simulink model "altitude_from_pitch_loop"  (Simulink 7.4)
settings: Solver=ode45  StartTime=0.0  StopTime=100  RelTol=1e-3
values from neighbouring files (symbols this model uses):
  a_theta1 = den(2)    [computeGains.m]    (also in compute_tf_model.m = -rho*Va_trim^2 * cbar^2 * S_wing /(4*P.Jy) * P.C_M_q)
  a_theta2 = num(3)    [computeGains.m]    (also in compute_tf_model.m = -rho*Va_trim^2*cbar*S_wing/2/P.Jy*C_M_alpha)
  a_theta3 = rho*Va_trim^2*cbar*S_wing/2/P.Jy*C_M_delta_e    [compute_tf_model.m]
  delta_e_max = P.delta_e_max    [computeGains.m]
  P = varargin{5}    [my_mav_dynamics.m]
settings Model: Creator=beard  LastModifiedBy=beard

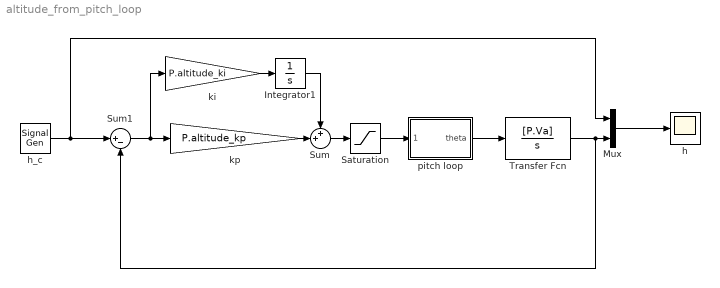
== system altitude_from_pitch_loop ==
  Integrator1 : Integrator
  Mux : Mux  Inputs=2
  Saturation : Saturate  UpperLimit=30*pi/180/P.K_theta_DC  LowerLimit=-30*pi/180/P.K_theta_DC  OutDataType=fixdt(1, 16)  OutScaling=2^0
  Sum : Sum  Inputs=++|  OutDataType=fixdt(1, 16)  OutScaling=2^0
  Sum1 : Sum  Inputs=|+-  OutDataType=fixdt(1, 16)  OutScaling=2^0
  Transfer Fcn : TransferFcn  Numerator=[P.Va]  Denominator=[1 0]
  h : Scope
      settings: TimeRange=100  YMin=-10  YMax=15
  h_c : SignalGenerator  WaveForm=square  Amplitude=5  Frequency=.02
  ki : Gain  Gain=P.altitude_ki  ParameterDataType=fixdt(1, 16)  ParameterScaling=2^0  OutDataType=fixdt(1, 16)  OutScaling=2^0
  kp : Gain  Gain=P.altitude_kp  ParameterDataType=fixdt(1, 16)  ParameterScaling=2^0  OutDataType=fixdt(1, 16)  OutScaling=2^0
  pitch loop : Subsystem
  wires:
  Sum/1 -> Saturation/1
  kp/1 -> Sum/2
  Sum1/1 -> kp/1, ki/1
  ki/1 -> Integrator1/1
  Integrator1/1 -> Sum/1
  h_c/1 -> Sum1/1, Mux/1
  Mux/1 -> h/1
  pitch loop/1(theta) -> Transfer Fcn/1
  Transfer Fcn/1 -> Mux/2, Sum1/2
  Saturation/1 -> pitch loop/1(theta_c)

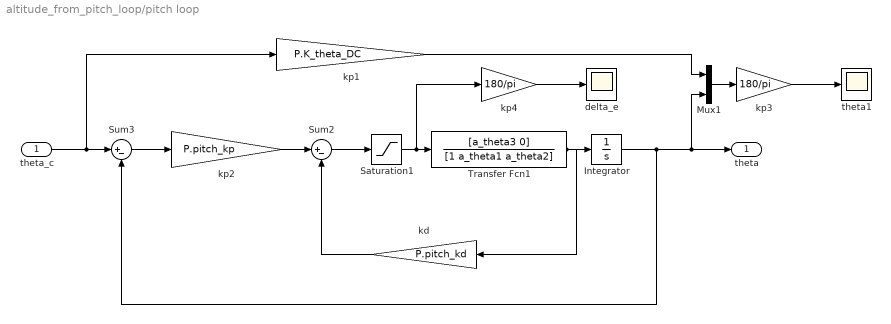
== system altitude_from_pitch_loop/pitch loop ==
  theta_c : Inport
  Integrator : Integrator
  Mux1 : Mux  Inputs=2
  Saturation1 : Saturate  UpperLimit=delta_e_max  LowerLimit=-delta_e_max  OutDataType=fixdt(1, 16)  OutScaling=2^0
  Sum2 : Sum  Inputs=|+-  OutDataType=fixdt(1, 16)  OutScaling=2^0
  Sum3 : Sum  Inputs=|+-  OutDataType=fixdt(1, 16)  OutScaling=2^0
  Transfer Fcn1 : TransferFcn  Numerator=[a_theta3 0]  Denominator=[1 a_theta1 a_theta2]
  delta_e : Scope
      settings: TimeRange=100  YMin=-10  YMax=15
  kd : Gain  Gain=P.pitch_kd  ParameterDataType=fixdt(1, 16)  ParameterScaling=2^0  OutDataType=fixdt(1, 16)  OutScaling=2^0
  kp1 : Gain  Gain=P.K_theta_DC  ParameterDataType=fixdt(1, 16)  ParameterScaling=2^0  OutDataType=fixdt(1, 16)  OutScaling=2^0
  kp2 : Gain  Gain=P.pitch_kp  ParameterDataType=fixdt(1, 16)  ParameterScaling=2^0  OutDataType=fixdt(1, 16)  OutScaling=2^0
  kp3 : Gain  Gain=180/pi  ParameterDataType=fixdt(1, 16)  ParameterScaling=2^0  OutDataType=fixdt(1, 16)  OutScaling=2^0
  kp4 : Gain  Gain=180/pi  ParameterDataType=fixdt(1, 16)  ParameterScaling=2^0  OutDataType=fixdt(1, 16)  OutScaling=2^0
  theta1 : Scope
      settings: TimeRange=100  YMin=-40  YMax=40  SaveName=ScopeData2
  theta : Outport
  wires:
  Transfer Fcn1/1 -> Integrator/1, kd/1
  Saturation1/1 -> Transfer Fcn1/1, kp4/1
  Sum2/1 -> Saturation1/1
  Sum3/1 -> kp2/1
  Integrator/1 -> Sum3/2, Mux1/2, theta/1
  theta_c/1 -> Sum3/1, kp1/1
  Mux1/1 -> kp3/1
  kp4/1 -> delta_e/1
  kp2/1 -> Sum2/1
  kd/1 -> Sum2/2
  kp3/1 -> theta1/1
  kp1/1 -> Mux1/1
